simulink model "SPWM_tiaozhi"  (R2024b)
settings: Solver=VariableStepAuto  StartTime=1  StopTime=20  RelTol=1e-5  AbsTol=1e-5
libraries: fl_lib x9, nesl_utility x8, spsControlledVoltageSourceLib x3, ee_lib x3, spsPermanentMagnetSynchronousMachineLib x1, simulink x1, sps_lib x1
settings Model: SimulationMode=accelerator  Creator=刘炳宏  LastModifiedBy=刘炳宏
settings DataIOCC: ReturnWorkspaceOutputs=off

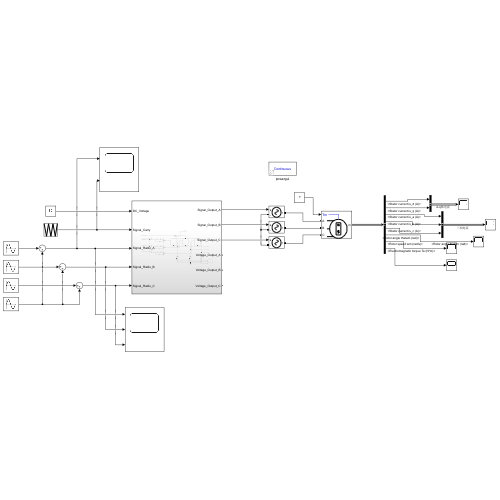
[thumbnail: Simulink's stored preview of the top-level diagram]
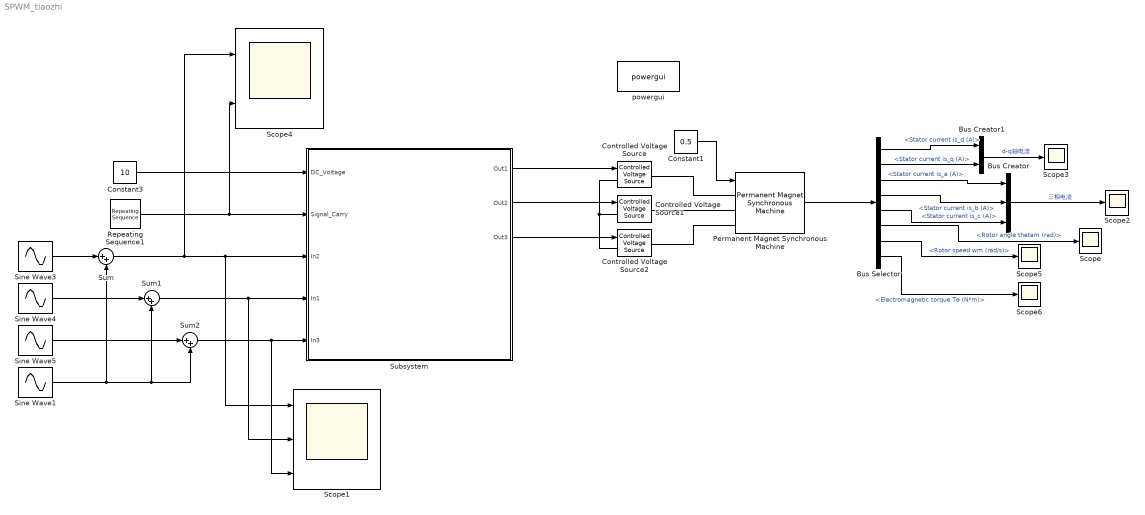
== system SPWM_tiaozhi ==
  Bus Creator : BusCreator  Inputs=3
  Bus Creator1 : BusCreator  Inputs=2
  Bus Selector : BusSelector  OutputSignals=Stator current is_d (A),Stator current is_q (A),Stator current is_a (A),Stator current is_b (A),Stator current is_c (A),Rotor angle thetam (rad),Rotor speed wm (rad/s),Electromagnetic torque Te (N*m)
  Constant1 : Constant  Value=0.5
  Constant3 : Constant  Value=10
  Controlled Voltage Source : spsControlledVoltageSourceLib/Controlled Voltage Source  Initialize=on  Source_Type=DC  Amplitude=0  Phase=0  Frequency=0  Measurements=None
  Controlled Voltage Source1 : spsControlledVoltageSourceLib/Controlled Voltage Source  Initialize=on  Source_Type=DC  Amplitude=0  Phase=0  Frequency=0  Measurements=None
  Controlled Voltage Source2 : spsControlledVoltageSourceLib/Controlled Voltage Source  Initialize=on  Source_Type=DC  Amplitude=0  Phase=0  Frequency=0  Measurements=None
  Permanent Magnet Synchronous Machine : spsPermanentMagnetSynchronousMachineLib/Permanent Magnet Synchronous Machine  NbPhases=3  FluxDistribution=Sinusoidal  RotorType=Round  MechanicalLoad=Torque Tm  PresetModel=No  ShowDetailedParameters=on  MeasurementBus=off  Resistance=0.18  Inductance=8.5e-3  dqInductances=[8.5e-3,8.5e-3]  La=8.5e-3  MachineConstant=Flux linkage established by magnets (V.s)  Flux=0.074147  VoltageCst=134.4878  TorqueCst=1.1122  Flat=120  Mechanical=[0.00062 0.0003505 10 0]  PolePairs=4  InitialConditions=[0,1, 0,0]  InitialConditions5ph=[0 0 0 0 0 0]  RefAngle=Aligned with phase A axis (original Park)  IterativeDiscreteModel=Trapezoidal non iterative  TsBlock=-1  TsPowergui=0
  Repeating Sequence1 : simulink/Sources/Repeating Sequence  rep_seq_t=[0,0.5/(5000),1/(5000)]  rep_seq_y=[1,-1,1]
  Scope{,2..3,5..6} (5 alike) : Scope
  Scope1 : Scope  NumInputPorts=3
  Scope4 : Scope  NumInputPorts=2
  Sine Wave1 : Sin  Amplitude=0.02*10  Frequency=6*3.14159*5*10  SampleTime=0
  Sine Wave3 : Sin  Amplitude=0.05*10  Frequency=2*3.14159*5*10  SampleTime=0
  Sine Wave4 : Sin  Amplitude=0.05*10  Frequency=2*3.14159*5*10  Phase=2*3.14159/3  SampleTime=0
  Sine Wave5 : Sin  Amplitude=0.05*10  Frequency=2*3.14159*5*10  Phase=-2*3.14159/3  SampleTime=0
  Subsystem : Subsystem
  Sum : Sum  Inputs=|++
  Sum1 : Sum  Inputs=|++
  Sum2 : Sum  Inputs=|++
  powergui : sps_lib/powergui  Priority=1  SimulationMode=Continuous  SampleTime=50e-6  frequency=60  Iterations=50  frequencyindice=0  Pbase=100e6  ErrMax=1e-4  UnitsV=kV  UnitsW=MW  buscounter=0  FunctionMessages=off  echomessages=off  EnableUseOfTLC=off  CurrentSourceSwitches=off  DisableSnubberDevices=off  DisableRonSwitches=off  DisableVfSwitches=off  DisplayEquations=off  AutomaticDiscreteSolvers=off  SolverType=Tustin/Backward Euler (TBE)  Interpol=off  ExternalGateDelay=off  methode=off  Ts=100  x0status=blocks  SPID=on  SwTol=0  HookPort=off  NonlinearTolerance=1e-4  nMaxIteration=100  ContinueOnMaxIteration=off  RestoreLinks=warning  ResistiveCurrentMeasurement=off  Frange=[0:2:500]  Ylog=off  Xlog=on  ShowGrid=off  save=off  variable=ZData  structure=0  ZoomFFT=off  StartTime=0.0  cycles=1  DisplayStyle=1  fundamental=60  FreqAxis=off  MaxFrequency=1000  frequencyindicesteady=1  RmsSteady=1  display=off
  wires:
  Repeating Sequence1/1 -> Scope4/2, Subsystem/2(Signal_Carry)
  Constant3/1 -> Subsystem/1(DC_Voltage)
  Sine Wave3/1 -> Sum/1
  Sum/1 -> Scope4/1, Scope1/1, Subsystem/3(In2)
  Sum1/1 -> Scope1/2, Subsystem/4(In1)
  Sine Wave4/1 -> Sum1/1
  Sine Wave1/1 -> Sum2/2, Sum1/2, Sum/2
  Sine Wave5/1 -> Sum2/1
  Sum2/1 -> Scope1/3, Subsystem/5(In3)
  Subsystem/1(Out1) -> Controlled Voltage Source/1
  Subsystem/3(Out3) -> Controlled Voltage Source2/1
  Subsystem/2(Out2) -> Controlled Voltage Source1/1
  Bus Selector/5 -> Bus Creator/3  "<Stator current is_c (A)>"
  Bus Selector/4 -> Bus Creator/2  "<Stator current is_b (A)>"
  Bus Selector/2 -> Bus Creator1/2  "<Stator current is_q (A)>"
  Bus Selector/1 -> Bus Creator1/1  "<Stator current is_d (A)>"
  Bus Creator1/1 -> Scope3/1  "d-q轴电流"
  Permanent Magnet Synchronous Machine/1 -> Bus Selector/1
  Bus Creator/1 -> Scope2/1  "三相电流"
  Bus Selector/3 -> Bus Creator/1  "<Stator current is_a (A)>"
  Bus Selector/6 -> Scope/1  "<Rotor angle thetam (rad)>"
  Bus Selector/7 -> Scope5/1  "<Rotor speed wm (rad/s)>"
  Bus Selector/8 -> Scope6/1  "<Electromagnetic torque Te (N*m)>"
  Constant1/1 -> Permanent Magnet Synchronous Machine/1
  connections:
  Controlled Voltage Source/LConn1 -- Controlled Voltage Source1/LConn1 -- Controlled Voltage Source2/LConn1
  Permanent Magnet Synchronous Machine/LConn2 -- Controlled Voltage Source1/RConn1
  Permanent Magnet Synchronous Machine/LConn1 -- Controlled Voltage Source/RConn1
  Permanent Magnet Synchronous Machine/LConn3 -- Controlled Voltage Source2/RConn1

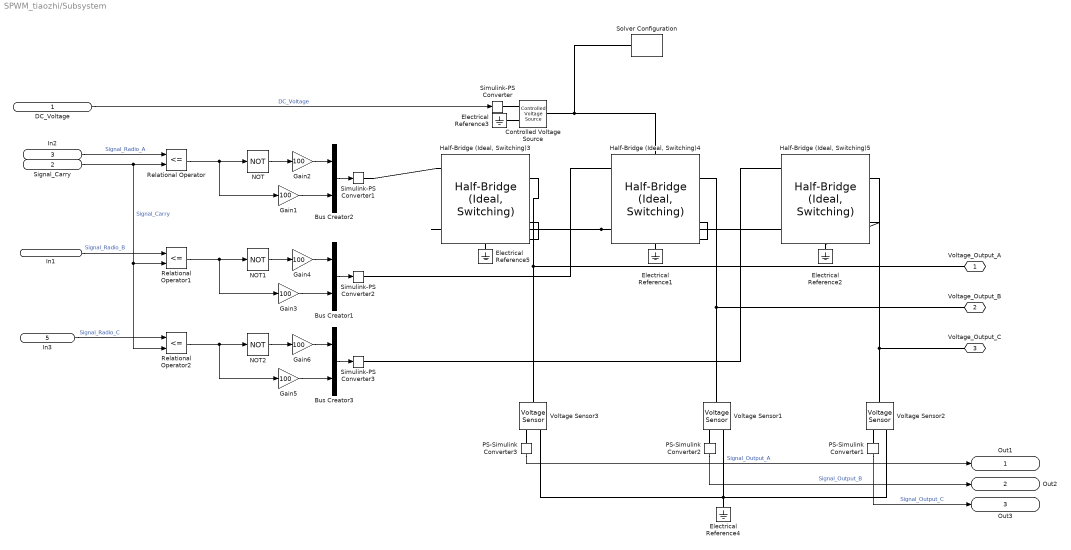
== system SPWM_tiaozhi/Subsystem ==
  DC_Voltage : Inport
  Signal_Carry : Inport  Port=2
  In2 : Inport  Port=3
  In1 : Inport  Port=4
  In3 : Inport  Port=5
  Bus Creator1 : BusCreator  Inputs=2
  Bus Creator2 : BusCreator  Inputs=2
  Bus Creator3 : BusCreator  Inputs=2
  Controlled Voltage Source : fl_lib/Electrical/Electrical Sources/Controlled Voltage Source
  Electrical Reference{1..5} (5 alike) : fl_lib/Electrical/Electrical Elements/Electrical Reference
  Gain{1..6} (6 alike) : Gain  Gain=100  OutDataTypeStr=double
  "Half-Bridge (Ideal, Switching)3" : ee_lib/Semiconductors & Converters/Half-Bridge (Ideal, Switching)  control_port=ee.enum.controlport.ps  device_type=ee.enum.converters.switches.mosfet  gto_Vgt=6 V  gto_Vgt_off=-1 V  gto_Ih=1 A  gto_thermal_loss_option=ee.enum.converters.thermalLossOption.constantvalues  gto_Vf=0.8 V  gto_Ron=0.001 Ohm  gto_Von_data=[0, .1, .6, .8, 1, 1.3, 1.6, 2, 2.4; 0, .1, .7, 1, 1.2, 1.5, 1.9, 2.4, 2.8] V  gto_Tj=[298.15, 398.15] K  gto_Iout_data=[0, .1, 1, 5, 10, 20, 40, 70, 100] A  igbt_Vth=6 V  igbt_thermal_loss_option=ee.enum.converters.thermalLossOption.constantvalues  igbt_Vf=0.8 V  igbt_Ron=0.001 Ohm  igbt_Von_data=[0, .1, .6, .8, 1, 1.3, 1.6, 2, 2.4; 0, .1, .7, 1, 1.2, 1.5, 1.9, 2.4, 2.8] V  igbt_Tj=[298.15, 398.15] K  igbt_Iout_data=[0, .1, 1, 5, 10, 20, 40, 70, 100] A  mosfet_Vth=2 V  mosfet_thermal_loss_option=ee.enum.converters.thermalLossOption.constantvalues  mosfet_Rds=0.01 Ohm  mosfet_Von_data=[0, 1.1, 1.3, 1.45, 1.75, 2.25, 2.7; 0, 1, 1.15, 1.35, 1.7, 2.35, 3] V  mosfet_Tj=[298.15, 398.15] K  mosfet_Iout_data=[0, 10, 50, 100, 200, 400, 600] A  Goff=1e-6 1/Ohm  gto_Eon_data=[0, .0024, .024, .12, .2, .48, 1.04, 2.16, 3.24; 0, .003, .03, .15, .25, .6, 1.3, 2.7, 4.05] * 1e-3 J  igbt_Eon_data=[0, .0024, .024, .12, .2, .48, 1.04, 2.16, 3.24; 0, .003, .03, .15, .25, .6, 1.3, 2.7, 4.05] * 1e-3 J  mosfet_Eon_data=[0, .29, 1.43, 2.86, 5.71, 13.14, 22.86; 0, .57, 2.63, 5.14, 10.29, 20.57, 30.29] * 1e-3 J  gto_Eoff_data=[0, .0007, .0066, .033, .066, .17, .33, .83, 1.5; 0, .001, .01, .05, .1, .25, .5, 1.2, 2.2] * 1e-3 J  igbt_Eoff_data=[0, .0007, .0066, .033, .066, .17, .33, .83, 1.5; 0, .001, .01, .05, .1, .25, .5, 1.2, 2.2] * 1e-3 J  mosfet_Eoff_data=[0, .21, 1.07, 2.14, 4.29, 9.86, 17.14; 0, .43, 1.97, 3.86, 7.71, 15.43, 22.71] * 1e-3 J  igbt_Eon_data_3D=[zeros(2, 9, 3)] J  mosfet_Eon_data_3D=[zeros(2, 7, 3)] J  igbt_Eoff_data_3D=[zeros(2, 9, 3)] J  mosfet_Eoff_data_3D=[zeros(2, 7, 3)] J  gto_Erec_data=[0, .0031, .021, .11, .21, .43, .99, 1.71, 3.078; 0, .0041, .043, .2, .39, .77, 1.54, 2.27, 4.08] * 1e-3 J  igbt_Erec_data=[0, .0031, .021, .11, .21, .43, .99, 1.71, 3.078; 0, .0041, .043, .2, .39, .77, 1.54, 2.27, 4.08] * 1e-3 J  mosfet_Erec_data=[0, .0031, .021, .11, .21, .43, .99; 0, .0041, .043, .2, .39, .77, 1.54] * 1e-3 J  gto_Tj_loss=[298.15, 398.15] K  igbt_Tj_loss=[298.15, 398.15] K  mosfet_Tj_loss=[298.15, 398.15] K  gto_Iout_data_loss=[0, .1, 1, 5, 10, 20, 40, 70, 100] A  igbt_Iout_data_loss=[0, .1, 1, 5, 10, 20, 40, 70, 100] A  mosfet_Iout_data_loss=[0, 10, 50, 100, 200, 400, 600] A  gto_Eon_scalar=22.86e-3 J  igbt_Eon_scalar=22.86e-3 J  mosfet_Eon_scalar=22.86e-3 J  gto_Eoff_scalar=17.14e-3 J  igbt_Eoff_scalar=17.14e-3 J  mosfet_Eoff_scalar=17.14e-3 J  gto_Erec_scalar=5.70e-3 J  igbt_Erec_scalar=5.70e-3 J  mosfet_Erec_scalar=5.70e-3 J  gto_Iout_scalar=600 A  igbt_Iout_scalar=600 A  mosfet_Iout_scalar=600 A  igbt_tabulateWithVce=false  mosfet_tabulateWithVds=false  igbt_Vce_loss=[0, 150, 300] V  mosfet_Vds_loss=[0, 150, 300] V  Voff=300 V  gto_Eoff_natural_commutation=10e-3 J  applySwLossToSupply=false  tauApplySwLoss=1e-3 s  diode_param=ee.enum.include.yes  diode_ModelType=ee.enum.converters.diodeModelType.pwl  diode_TableType=ee.enum.diode.tableType.IfMat  diode_ReverseIVType=ee.enum.diode.diodeReverseIV.constant  diode_IfMat=[.07, .12, .19, 1.75, 4.24, 7.32, 11.2; .16, .3, .72, 2.14, 4.02, 6.35, 9.12] A  diode_VfMat=[.9, 1.15, 1.25, 1.5, 1.75, 2.17, 2.6, 2.85; .58, .68, .75, 1.1, 1.38, 1.77, 2.27, 2.7] V  diode_TjVec=[25, 125] degC  diode_VfVec=[.5, .7, .9, 1.3, 1.7, 2.1, 2.5] V  diode_IfVec=[.1, .2, .5, 1, 2, 4, 7, 10] A  diode_IrMat=[1e-06, 2e-06, 5e-06, 1e-05, 2.5e-05, 5e-05, .0001; 2e-06, 5e-06, 1e-05, 4e-05, 8e-05, .0002, .0005] A  diode_VrMat=[10, 100, 200, 250, 300, 325, 350; 10, 70, 160, 220, 270, 300, 320] V  diode_VrVec=[10, 20, 40, 50, 70, 80, 100] V  diode_IrVec=[1e-06, 2e-06, 5e-06, 1e-05, 2e-05, 5e-05, .0001] A  diode_Vf=0.8 V  diode_Ron=0.001 Ohm  diode_Goff=1e-5 1/Ohm  separateThermalPort=false  separateThermalPortsForDiodes=false  thermal_network_parameterization=ee.enum.thermalNetworkTopology.external  thermal_mass_parameterization=ee.enum.thermalNetwork.timeconstant  Rth=[.03, .2] K/W  Rth_Cauer=[.03, .1, .2] K/W  Rth_Foster=[.08, .14, .22, .16] K/W  thermal_mass=[3, 25] J/K  thermal_mass_Cauer=[3, 10, 25] J/K  thermal_mass_Foster=[.001, .005, .05, .5] J/K  thermal_time_constant=[.1, 5] s  thermal_time_constant_Cauer=[.1, 1, 5] s  thermal_time_constant_Foster=[7e-05, .0007, .01, .08] s  thermal_mass_initial_temperatures=[25, 25] degC  thermal_mass_initial_temperatures_Cauer=[25, 25, 25] degC  junction_thermal_mass=0.1 J/K  Tvec_initial_Foster=[25, 25, 25, 25] degC  RthDiode=[.03, .2] K/W  RthCauerDiode=[.03, .1, .2] K/W  RthFosterDiode=[.08, .14, .22, .16] K/W  ThermalMassDiode=[3, 25] J/K  ThermalMassCauerDiode=[3, 10, 25] J/K  ThermalMassFosterDiode=[.001, .005, .05, .5] J/K  ThermalTauDiode=[.1, 5] s  ThermalTauCauerDiode=[.1, 1, 5] s  ThermalTauFosterDiode=[7e-05, .0007, .01, .08] s  ThermalMassInitTempDiode=[25, 25] degC  ThermalMassInitTempCauerDiode=[25, 25, 25] degC  JunctionThermalMassDiode=0.1 J/K  TVecInitialFosterDiode=[25, 25, 25, 25] degC  junction_temperature_specify=off  junction_temperature_priority=None  junction_temperature=25 degC  junction_temperature_nominal_specify=off  junction_temperature_nominal_value=1  junction_temperature_nominal_unit=degC  upperSwitchTemp_specify=off  upperSwitchTemp_priority=None  upperSwitchTemp=25 degC  upperSwitchTemp_nominal_specify=off  upperSwitchTemp_nominal_value=1  upperSwitchTemp_nominal_unit=degC  lowerSwitchTemp_specify=off  lowerSwitchTemp_priority=None  lowerSwitchTemp=25 degC  lowerSwitchTemp_nominal_specify=off  lowerSwitchTemp_nominal_value=1  lowerSwitchTemp_nominal_unit=degC  upperDiodeTemp_specify=off  upperDiodeTemp_priority=None  upperDiodeTemp=25 degC  upperDiodeTemp_nominal_specify=off  upperDiodeTemp_nominal_value=1  upperDiodeTemp_nominal_unit=degC  lowerDiodeTemp_specify=off  lowerDiodeTemp_priority=None  lowerDiodeTemp=25 degC  lowerDiodeTemp_nominal_specify=off  lowerDiodeTemp_nominal_value=1  lowerDiodeTemp_nominal_unit=degC
      settings: InternalSimscapePortConfiguration="{\"Bottom\":[{\"id\":\"n\",\"label\":\"-\",\"type\":\"foundation.electrical.electrical\"}],\"Left\":[{\"id\":\"G\",\"label\":\"G\",\"type\":\"input\"},{\"id\":\"H\",\"label\":\"H\",\"type\":\"foundation.thermal.thermal\"}],\"Right\":[{\"id\":\"o\",\"label\":\"o\",\"type\":\"foundation.electrical.electrical\"}],\"Top\":[{\"id\":\"p\",\"label\":\"+\",\"type\":\"foundation.electrical.electrical\"}]}"
  "Half-Bridge (Ideal, Switching)4" : ee_lib/Semiconductors & Converters/Half-Bridge (Ideal, Switching)  control_port=ee.enum.controlport.ps  device_type=ee.enum.converters.switches.mosfet  gto_Vgt=6 V  gto_Vgt_off=-1 V  gto_Ih=1 A  gto_thermal_loss_option=ee.enum.converters.thermalLossOption.constantvalues  gto_Vf=0.8 V  gto_Ron=0.001 Ohm  gto_Von_data=[0, .1, .6, .8, 1, 1.3, 1.6, 2, 2.4; 0, .1, .7, 1, 1.2, 1.5, 1.9, 2.4, 2.8] V  gto_Tj=[298.15, 398.15] K  gto_Iout_data=[0, .1, 1, 5, 10, 20, 40, 70, 100] A  igbt_Vth=6 V  igbt_thermal_loss_option=ee.enum.converters.thermalLossOption.constantvalues  igbt_Vf=0.8 V  igbt_Ron=0.001 Ohm  igbt_Von_data=[0, .1, .6, .8, 1, 1.3, 1.6, 2, 2.4; 0, .1, .7, 1, 1.2, 1.5, 1.9, 2.4, 2.8] V  igbt_Tj=[298.15, 398.15] K  igbt_Iout_data=[0, .1, 1, 5, 10, 20, 40, 70, 100] A  mosfet_Vth=2 V  mosfet_thermal_loss_option=ee.enum.converters.thermalLossOption.constantvalues  mosfet_Rds=0.01 Ohm  mosfet_Von_data=[0, 1.1, 1.3, 1.45, 1.75, 2.25, 2.7; 0, 1, 1.15, 1.35, 1.7, 2.35, 3] V  mosfet_Tj=[298.15, 398.15] K  mosfet_Iout_data=[0, 10, 50, 100, 200, 400, 600] A  Goff=1e-6 1/Ohm  gto_Eon_data=[0, .0024, .024, .12, .2, .48, 1.04, 2.16, 3.24; 0, .003, .03, .15, .25, .6, 1.3, 2.7, 4.05] * 1e-3 J  igbt_Eon_data=[0, .0024, .024, .12, .2, .48, 1.04, 2.16, 3.24; 0, .003, .03, .15, .25, .6, 1.3, 2.7, 4.05] * 1e-3 J  mosfet_Eon_data=[0, .29, 1.43, 2.86, 5.71, 13.14, 22.86; 0, .57, 2.63, 5.14, 10.29, 20.57, 30.29] * 1e-3 J  gto_Eoff_data=[0, .0007, .0066, .033, .066, .17, .33, .83, 1.5; 0, .001, .01, .05, .1, .25, .5, 1.2, 2.2] * 1e-3 J  igbt_Eoff_data=[0, .0007, .0066, .033, .066, .17, .33, .83, 1.5; 0, .001, .01, .05, .1, .25, .5, 1.2, 2.2] * 1e-3 J  mosfet_Eoff_data=[0, .21, 1.07, 2.14, 4.29, 9.86, 17.14; 0, .43, 1.97, 3.86, 7.71, 15.43, 22.71] * 1e-3 J  igbt_Eon_data_3D=[zeros(2, 9, 3)] J  mosfet_Eon_data_3D=[zeros(2, 7, 3)] J  igbt_Eoff_data_3D=[zeros(2, 9, 3)] J  mosfet_Eoff_data_3D=[zeros(2, 7, 3)] J  gto_Erec_data=[0, .0031, .021, .11, .21, .43, .99, 1.71, 3.078; 0, .0041, .043, .2, .39, .77, 1.54, 2.27, 4.08] * 1e-3 J  igbt_Erec_data=[0, .0031, .021, .11, .21, .43, .99, 1.71, 3.078; 0, .0041, .043, .2, .39, .77, 1.54, 2.27, 4.08] * 1e-3 J  mosfet_Erec_data=[0, .0031, .021, .11, .21, .43, .99; 0, .0041, .043, .2, .39, .77, 1.54] * 1e-3 J  gto_Tj_loss=[298.15, 398.15] K  igbt_Tj_loss=[298.15, 398.15] K  mosfet_Tj_loss=[298.15, 398.15] K  gto_Iout_data_loss=[0, .1, 1, 5, 10, 20, 40, 70, 100] A  igbt_Iout_data_loss=[0, .1, 1, 5, 10, 20, 40, 70, 100] A  mosfet_Iout_data_loss=[0, 10, 50, 100, 200, 400, 600] A  gto_Eon_scalar=22.86e-3 J  igbt_Eon_scalar=22.86e-3 J  mosfet_Eon_scalar=22.86e-3 J  gto_Eoff_scalar=17.14e-3 J  igbt_Eoff_scalar=17.14e-3 J  mosfet_Eoff_scalar=17.14e-3 J  gto_Erec_scalar=5.70e-3 J  igbt_Erec_scalar=5.70e-3 J  mosfet_Erec_scalar=5.70e-3 J  gto_Iout_scalar=600 A  igbt_Iout_scalar=600 A  mosfet_Iout_scalar=600 A  igbt_tabulateWithVce=false  mosfet_tabulateWithVds=false  igbt_Vce_loss=[0, 150, 300] V  mosfet_Vds_loss=[0, 150, 300] V  Voff=300 V  gto_Eoff_natural_commutation=10e-3 J  applySwLossToSupply=false  tauApplySwLoss=1e-3 s  diode_param=ee.enum.include.yes  diode_ModelType=ee.enum.converters.diodeModelType.pwl  diode_TableType=ee.enum.diode.tableType.IfMat  diode_ReverseIVType=ee.enum.diode.diodeReverseIV.constant  diode_IfMat=[.07, .12, .19, 1.75, 4.24, 7.32, 11.2; .16, .3, .72, 2.14, 4.02, 6.35, 9.12] A  diode_VfMat=[.9, 1.15, 1.25, 1.5, 1.75, 2.17, 2.6, 2.85; .58, .68, .75, 1.1, 1.38, 1.77, 2.27, 2.7] V  diode_TjVec=[25, 125] degC  diode_VfVec=[.5, .7, .9, 1.3, 1.7, 2.1, 2.5] V  diode_IfVec=[.1, .2, .5, 1, 2, 4, 7, 10] A  diode_IrMat=[1e-06, 2e-06, 5e-06, 1e-05, 2.5e-05, 5e-05, .0001; 2e-06, 5e-06, 1e-05, 4e-05, 8e-05, .0002, .0005] A  diode_VrMat=[10, 100, 200, 250, 300, 325, 350; 10, 70, 160, 220, 270, 300, 320] V  diode_VrVec=[10, 20, 40, 50, 70, 80, 100] V  diode_IrVec=[1e-06, 2e-06, 5e-06, 1e-05, 2e-05, 5e-05, .0001] A  diode_Vf=0.8 V  diode_Ron=0.001 Ohm  diode_Goff=1e-5 1/Ohm  separateThermalPort=false  separateThermalPortsForDiodes=false  thermal_network_parameterization=ee.enum.thermalNetworkTopology.external  thermal_mass_parameterization=ee.enum.thermalNetwork.timeconstant  Rth=[.03, .2] K/W  Rth_Cauer=[.03, .1, .2] K/W  Rth_Foster=[.08, .14, .22, .16] K/W  thermal_mass=[3, 25] J/K  thermal_mass_Cauer=[3, 10, 25] J/K  thermal_mass_Foster=[.001, .005, .05, .5] J/K  thermal_time_constant=[.1, 5] s  thermal_time_constant_Cauer=[.1, 1, 5] s  thermal_time_constant_Foster=[7e-05, .0007, .01, .08] s  thermal_mass_initial_temperatures=[25, 25] degC  thermal_mass_initial_temperatures_Cauer=[25, 25, 25] degC  junction_thermal_mass=0.1 J/K  Tvec_initial_Foster=[25, 25, 25, 25] degC  RthDiode=[.03, .2] K/W  RthCauerDiode=[.03, .1, .2] K/W  RthFosterDiode=[.08, .14, .22, .16] K/W  ThermalMassDiode=[3, 25] J/K  ThermalMassCauerDiode=[3, 10, 25] J/K  ThermalMassFosterDiode=[.001, .005, .05, .5] J/K  ThermalTauDiode=[.1, 5] s  ThermalTauCauerDiode=[.1, 1, 5] s  ThermalTauFosterDiode=[7e-05, .0007, .01, .08] s  ThermalMassInitTempDiode=[25, 25] degC  ThermalMassInitTempCauerDiode=[25, 25, 25] degC  JunctionThermalMassDiode=0.1 J/K  TVecInitialFosterDiode=[25, 25, 25, 25] degC  junction_temperature_specify=off  junction_temperature_priority=None  junction_temperature=25 degC  junction_temperature_nominal_specify=off  junction_temperature_nominal_value=1  junction_temperature_nominal_unit=degC  upperSwitchTemp_specify=off  upperSwitchTemp_priority=None  upperSwitchTemp=25 degC  upperSwitchTemp_nominal_specify=off  upperSwitchTemp_nominal_value=1  upperSwitchTemp_nominal_unit=degC  lowerSwitchTemp_specify=off  lowerSwitchTemp_priority=None  lowerSwitchTemp=25 degC  lowerSwitchTemp_nominal_specify=off  lowerSwitchTemp_nominal_value=1  lowerSwitchTemp_nominal_unit=degC  upperDiodeTemp_specify=off  upperDiodeTemp_priority=None  upperDiodeTemp=25 degC  upperDiodeTemp_nominal_specify=off  upperDiodeTemp_nominal_value=1  upperDiodeTemp_nominal_unit=degC  lowerDiodeTemp_specify=off  lowerDiodeTemp_priority=None  lowerDiodeTemp=25 degC  lowerDiodeTemp_nominal_specify=off  lowerDiodeTemp_nominal_value=1  lowerDiodeTemp_nominal_unit=degC
      settings: InternalSimscapePortConfiguration="{\"Bottom\":[{\"id\":\"n\",\"label\":\"-\",\"type\":\"foundation.electrical.electrical\"}],\"Left\":[{\"id\":\"G\",\"label\":\"G\",\"type\":\"input\"},{\"id\":\"H\",\"label\":\"H\",\"type\":\"foundation.thermal.thermal\"}],\"Right\":[{\"id\":\"o\",\"label\":\"o\",\"type\":\"foundation.electrical.electrical\"}],\"Top\":[{\"id\":\"p\",\"label\":\"+\",\"type\":\"foundation.electrical.electrical\"}]}"
  "Half-Bridge (Ideal, Switching)5" : ee_lib/Semiconductors & Converters/Half-Bridge (Ideal, Switching)  control_port=ee.enum.controlport.ps  device_type=ee.enum.converters.switches.mosfet  gto_Vgt=6 V  gto_Vgt_off=-1 V  gto_Ih=1 A  gto_thermal_loss_option=ee.enum.converters.thermalLossOption.constantvalues  gto_Vf=0.8 V  gto_Ron=0.001 Ohm  gto_Von_data=[0, .1, .6, .8, 1, 1.3, 1.6, 2, 2.4; 0, .1, .7, 1, 1.2, 1.5, 1.9, 2.4, 2.8] V  gto_Tj=[298.15, 398.15] K  gto_Iout_data=[0, .1, 1, 5, 10, 20, 40, 70, 100] A  igbt_Vth=6 V  igbt_thermal_loss_option=ee.enum.converters.thermalLossOption.constantvalues  igbt_Vf=0.8 V  igbt_Ron=0.001 Ohm  igbt_Von_data=[0, .1, .6, .8, 1, 1.3, 1.6, 2, 2.4; 0, .1, .7, 1, 1.2, 1.5, 1.9, 2.4, 2.8] V  igbt_Tj=[298.15, 398.15] K  igbt_Iout_data=[0, .1, 1, 5, 10, 20, 40, 70, 100] A  mosfet_Vth=2 V  mosfet_thermal_loss_option=ee.enum.converters.thermalLossOption.constantvalues  mosfet_Rds=0.01 Ohm  mosfet_Von_data=[0, 1.1, 1.3, 1.45, 1.75, 2.25, 2.7; 0, 1, 1.15, 1.35, 1.7, 2.35, 3] V  mosfet_Tj=[298.15, 398.15] K  mosfet_Iout_data=[0, 10, 50, 100, 200, 400, 600] A  Goff=1e-6 1/Ohm  gto_Eon_data=[0, .0024, .024, .12, .2, .48, 1.04, 2.16, 3.24; 0, .003, .03, .15, .25, .6, 1.3, 2.7, 4.05] * 1e-3 J  igbt_Eon_data=[0, .0024, .024, .12, .2, .48, 1.04, 2.16, 3.24; 0, .003, .03, .15, .25, .6, 1.3, 2.7, 4.05] * 1e-3 J  mosfet_Eon_data=[0, .29, 1.43, 2.86, 5.71, 13.14, 22.86; 0, .57, 2.63, 5.14, 10.29, 20.57, 30.29] * 1e-3 J  gto_Eoff_data=[0, .0007, .0066, .033, .066, .17, .33, .83, 1.5; 0, .001, .01, .05, .1, .25, .5, 1.2, 2.2] * 1e-3 J  igbt_Eoff_data=[0, .0007, .0066, .033, .066, .17, .33, .83, 1.5; 0, .001, .01, .05, .1, .25, .5, 1.2, 2.2] * 1e-3 J  mosfet_Eoff_data=[0, .21, 1.07, 2.14, 4.29, 9.86, 17.14; 0, .43, 1.97, 3.86, 7.71, 15.43, 22.71] * 1e-3 J  igbt_Eon_data_3D=[zeros(2, 9, 3)] J  mosfet_Eon_data_3D=[zeros(2, 7, 3)] J  igbt_Eoff_data_3D=[zeros(2, 9, 3)] J  mosfet_Eoff_data_3D=[zeros(2, 7, 3)] J  gto_Erec_data=[0, .0031, .021, .11, .21, .43, .99, 1.71, 3.078; 0, .0041, .043, .2, .39, .77, 1.54, 2.27, 4.08] * 1e-3 J  igbt_Erec_data=[0, .0031, .021, .11, .21, .43, .99, 1.71, 3.078; 0, .0041, .043, .2, .39, .77, 1.54, 2.27, 4.08] * 1e-3 J  mosfet_Erec_data=[0, .0031, .021, .11, .21, .43, .99; 0, .0041, .043, .2, .39, .77, 1.54] * 1e-3 J  gto_Tj_loss=[298.15, 398.15] K  igbt_Tj_loss=[298.15, 398.15] K  mosfet_Tj_loss=[298.15, 398.15] K  gto_Iout_data_loss=[0, .1, 1, 5, 10, 20, 40, 70, 100] A  igbt_Iout_data_loss=[0, .1, 1, 5, 10, 20, 40, 70, 100] A  mosfet_Iout_data_loss=[0, 10, 50, 100, 200, 400, 600] A  gto_Eon_scalar=22.86e-3 J  igbt_Eon_scalar=22.86e-3 J  mosfet_Eon_scalar=22.86e-3 J  gto_Eoff_scalar=17.14e-3 J  igbt_Eoff_scalar=17.14e-3 J  mosfet_Eoff_scalar=17.14e-3 J  gto_Erec_scalar=5.70e-3 J  igbt_Erec_scalar=5.70e-3 J  mosfet_Erec_scalar=5.70e-3 J  gto_Iout_scalar=600 A  igbt_Iout_scalar=600 A  mosfet_Iout_scalar=600 A  igbt_tabulateWithVce=false  mosfet_tabulateWithVds=false  igbt_Vce_loss=[0, 150, 300] V  mosfet_Vds_loss=[0, 150, 300] V  Voff=300 V  gto_Eoff_natural_commutation=10e-3 J  applySwLossToSupply=false  tauApplySwLoss=1e-3 s  diode_param=ee.enum.include.yes  diode_ModelType=ee.enum.converters.diodeModelType.pwl  diode_TableType=ee.enum.diode.tableType.IfMat  diode_ReverseIVType=ee.enum.diode.diodeReverseIV.constant  diode_IfMat=[.07, .12, .19, 1.75, 4.24, 7.32, 11.2; .16, .3, .72, 2.14, 4.02, 6.35, 9.12] A  diode_VfMat=[.9, 1.15, 1.25, 1.5, 1.75, 2.17, 2.6, 2.85; .58, .68, .75, 1.1, 1.38, 1.77, 2.27, 2.7] V  diode_TjVec=[25, 125] degC  diode_VfVec=[.5, .7, .9, 1.3, 1.7, 2.1, 2.5] V  diode_IfVec=[.1, .2, .5, 1, 2, 4, 7, 10] A  diode_IrMat=[1e-06, 2e-06, 5e-06, 1e-05, 2.5e-05, 5e-05, .0001; 2e-06, 5e-06, 1e-05, 4e-05, 8e-05, .0002, .0005] A  diode_VrMat=[10, 100, 200, 250, 300, 325, 350; 10, 70, 160, 220, 270, 300, 320] V  diode_VrVec=[10, 20, 40, 50, 70, 80, 100] V  diode_IrVec=[1e-06, 2e-06, 5e-06, 1e-05, 2e-05, 5e-05, .0001] A  diode_Vf=0.8 V  diode_Ron=0.001 Ohm  diode_Goff=1e-5 1/Ohm  separateThermalPort=false  separateThermalPortsForDiodes=false  thermal_network_parameterization=ee.enum.thermalNetworkTopology.external  thermal_mass_parameterization=ee.enum.thermalNetwork.timeconstant  Rth=[.03, .2] K/W  Rth_Cauer=[.03, .1, .2] K/W  Rth_Foster=[.08, .14, .22, .16] K/W  thermal_mass=[3, 25] J/K  thermal_mass_Cauer=[3, 10, 25] J/K  thermal_mass_Foster=[.001, .005, .05, .5] J/K  thermal_time_constant=[.1, 5] s  thermal_time_constant_Cauer=[.1, 1, 5] s  thermal_time_constant_Foster=[7e-05, .0007, .01, .08] s  thermal_mass_initial_temperatures=[25, 25] degC  thermal_mass_initial_temperatures_Cauer=[25, 25, 25] degC  junction_thermal_mass=0.1 J/K  Tvec_initial_Foster=[25, 25, 25, 25] degC  RthDiode=[.03, .2] K/W  RthCauerDiode=[.03, .1, .2] K/W  RthFosterDiode=[.08, .14, .22, .16] K/W  ThermalMassDiode=[3, 25] J/K  ThermalMassCauerDiode=[3, 10, 25] J/K  ThermalMassFosterDiode=[.001, .005, .05, .5] J/K  ThermalTauDiode=[.1, 5] s  ThermalTauCauerDiode=[.1, 1, 5] s  ThermalTauFosterDiode=[7e-05, .0007, .01, .08] s  ThermalMassInitTempDiode=[25, 25] degC  ThermalMassInitTempCauerDiode=[25, 25, 25] degC  JunctionThermalMassDiode=0.1 J/K  TVecInitialFosterDiode=[25, 25, 25, 25] degC  junction_temperature_specify=off  junction_temperature_priority=None  junction_temperature=25 degC  junction_temperature_nominal_specify=off  junction_temperature_nominal_value=1  junction_temperature_nominal_unit=degC  upperSwitchTemp_specify=off  upperSwitchTemp_priority=None  upperSwitchTemp=25 degC  upperSwitchTemp_nominal_specify=off  upperSwitchTemp_nominal_value=1  upperSwitchTemp_nominal_unit=degC  lowerSwitchTemp_specify=off  lowerSwitchTemp_priority=None  lowerSwitchTemp=25 degC  lowerSwitchTemp_nominal_specify=off  lowerSwitchTemp_nominal_value=1  lowerSwitchTemp_nominal_unit=degC  upperDiodeTemp_specify=off  upperDiodeTemp_priority=None  upperDiodeTemp=25 degC  upperDiodeTemp_nominal_specify=off  upperDiodeTemp_nominal_value=1  upperDiodeTemp_nominal_unit=degC  lowerDiodeTemp_specify=off  lowerDiodeTemp_priority=None  lowerDiodeTemp=25 degC  lowerDiodeTemp_nominal_specify=off  lowerDiodeTemp_nominal_value=1  lowerDiodeTemp_nominal_unit=degC
      settings: InternalSimscapePortConfiguration="{\"Bottom\":[{\"id\":\"n\",\"label\":\"-\",\"type\":\"foundation.electrical.electrical\"}],\"Left\":[{\"id\":\"G\",\"label\":\"G\",\"type\":\"input\"},{\"id\":\"H\",\"label\":\"H\",\"type\":\"foundation.thermal.thermal\"}],\"Right\":[{\"id\":\"o\",\"label\":\"o\",\"type\":\"foundation.electrical.electrical\"}],\"Top\":[{\"id\":\"p\",\"label\":\"+\",\"type\":\"foundation.electrical.electrical\"}]}"
  NOT : Logic  Operator=NOT  IconShape=distinctive  AllPortsSameDT=off  OutDataTypeStr=boolean
  NOT1 : Logic  Operator=NOT  IconShape=distinctive  AllPortsSameDT=off  OutDataTypeStr=boolean
  NOT2 : Logic  Operator=NOT  IconShape=distinctive  AllPortsSameDT=off  OutDataTypeStr=boolean
  PS-Simulink Converter1 : nesl_utility/PS-Simulink Converter  PhysicalDomain=network_engine_domain  SubClassName=ps_output  LeftPortType=input  RightPortType=output  PseudoPeriodic=off  Frequencies=[]  VectorFormat=inherit  Unit=inherit  AffineConversion=off
  PS-Simulink Converter2 : nesl_utility/PS-Simulink Converter  PhysicalDomain=network_engine_domain  SubClassName=ps_output  LeftPortType=input  RightPortType=output  PseudoPeriodic=off  Frequencies=[]  VectorFormat=inherit  Unit=inherit  AffineConversion=off
  PS-Simulink Converter3 : nesl_utility/PS-Simulink Converter  PhysicalDomain=network_engine_domain  SubClassName=ps_output  LeftPortType=input  RightPortType=output  PseudoPeriodic=off  Frequencies=[]  VectorFormat=inherit  Unit=inherit  AffineConversion=off
  Relational Operator : RelationalOperator  Operator=<=  OutDataTypeStr=boolean  RndMeth=Simplest  InputSameDT=off
  Relational Operator1 : RelationalOperator  Operator=<=  OutDataTypeStr=boolean  RndMeth=Simplest  InputSameDT=off
  Relational Operator2 : RelationalOperator  Operator=<=  OutDataTypeStr=boolean  RndMeth=Simplest  InputSameDT=off
  Simulink-PS Converter{,1..3} (4 alike) : nesl_utility/Simulink-PS Converter  PhysicalDomain=network_engine_domain  SubClassName=ps_input  LeftPortType=input  RightPortType=output  PseudoPeriodic=off  Frequencies=[]  NoiseDistribution=none  NoiseParameters=[]  Unit=1  AffineConversion=off  FilteringAndDerivatives=provide  SimscapeFilterOrder=1  InputFilterTimeConstant=0.001  UdotUserProvided=0
  Solver Configuration : nesl_utility/Solver Configuration  PhysicalDomain=network_engine_domain  SubClassName=solver  LeftPortType=input  RightPortType=generic  Tones=[]  Harmonics=[]  SimulateNoise=off  Profile=off  UseLocalSampling=off  EnableSwitchedLinearOptims=on  FrequencyDomain=off  UseCCode=off  RelTol=0.001  AbsTol=0.001  MinStep=1e-09  ToWorkspace=off  RevertToSquareIcSolve=off  NumHomotopyIterations=100  PhasorMode=off  PhasorModeNumHarmonics=1  ConsistencySolver=NEWTON_XTOL_AFTER_FTOL  IndexReductionMethod=DerivativeReplacement  DoDC=off  ResidualTolerance=1e-09  ConsistencyTolSource=GLOBAL  ConsistencyAbsTol=0.001  ConsistencyRelTol=0.001  ConsistencyTolFactor=0.001  UseLocalSolver=off  LocalSolverChoice=NE_BACKWARD_EULER_ADVANCER  ResolveIndetEquations=on  FunctionEvalNumThread=1  LocalSolverSampleTime=0.001  DoFixedCost=off  MaxNonlinIter=3  MaxModeIter=2  ComputeImpulses=off  ImpulseIterations=2  LinearAlgebra=auto  LinearAlgebraNumThread=0  EquationFormulation=NE_TIME_EF  DelaysMemoryBudget=1024  AutomaticFiltering=on  FilteringTimeConstant=0.001  PartitionStorageMethod=AS_NEEDED  PartitionMemoryBudget=1024  PartitionMethod=ROBUST  MultibodyUseLocalSolver=off  MultibodyLocalSolverChoice=ODE1  MultibodyLocalSolverSampleTime=0.001
  Voltage Sensor1 : fl_lib/Electrical/Electrical Sensors/Voltage Sensor
  Voltage Sensor2 : fl_lib/Electrical/Electrical Sensors/Voltage Sensor
  Voltage Sensor3 : fl_lib/Electrical/Electrical Sensors/Voltage Sensor
  Voltage_Output_A : PMIOPort  Side=Right
  Voltage_Output_B : PMIOPort  Port=2  Side=Right
  Voltage_Output_C : PMIOPort  Port=3  Side=Right
  Out1 : Outport
  Out2 : Outport  Port=2
  Out3 : Outport  Port=3
  wires:
  DC_Voltage/1 -> Simulink-PS Converter/1  "DC_Voltage"
  NOT/1 -> Gain2/1
  Relational Operator/1 -> Gain1/1, NOT/1
  Gain2/1 -> Bus Creator2/1
  Gain1/1 -> Bus Creator2/2
  Bus Creator2/1 -> Simulink-PS Converter1/1
  Signal_Carry/1 -> Relational Operator1/2, Relational Operator2/2, Relational Operator/2  "Signal_Carry"
  In2/1 -> Relational Operator/1  "Signal_Radio_A"
  Relational Operator1/1 -> Gain3/1, NOT1/1
  NOT1/1 -> Gain4/1
  Gain4/1 -> Bus Creator1/1
  Bus Creator1/1 -> Simulink-PS Converter2/1
  Gain3/1 -> Bus Creator1/2
  Relational Operator2/1 -> Gain5/1, NOT2/1
  NOT2/1 -> Gain6/1
  Gain6/1 -> Bus Creator3/1
  Bus Creator3/1 -> Simulink-PS Converter3/1
  Gain5/1 -> Bus Creator3/2
  In1/1 -> Relational Operator1/1  "Signal_Radio_B"
  In3/1 -> Relational Operator2/1  "Signal_Radio_C"
  PS-Simulink Converter3/1 -> Out1/1  "Signal_Output_A"
  PS-Simulink Converter2/1 -> Out2/1  "Signal_Output_B"
  PS-Simulink Converter1/1 -> Out3/1  "Signal_Output_C"
  connections:
  Electrical Reference5/LConn1 -- "Half-Bridge (Ideal, Switching)3"/RConn2
  Electrical Reference1/LConn1 -- "Half-Bridge (Ideal, Switching)4"/RConn2
  "Half-Bridge (Ideal, Switching)5"/RConn2 -- Electrical Reference2/LConn1
  "Half-Bridge (Ideal, Switching)3"/LConn3 -- Solver Configuration/RConn1 -- Controlled Voltage Source/LConn1 -- "Half-Bridge (Ideal, Switching)5"/LConn3 -- "Half-Bridge (Ideal, Switching)4"/LConn3
  Electrical Reference3/LConn1 -- Controlled Voltage Source/RConn2
  Simulink-PS Converter/RConn1 -- Controlled Voltage Source/RConn1
  Simulink-PS Converter1/RConn1 -- "Half-Bridge (Ideal, Switching)3"/LConn1
  Simulink-PS Converter2/RConn1 -- "Half-Bridge (Ideal, Switching)4"/LConn1
  Simulink-PS Converter3/RConn1 -- "Half-Bridge (Ideal, Switching)5"/LConn1
  Voltage Sensor3/LConn1 -- Voltage_Output_A/RConn1 -- "Half-Bridge (Ideal, Switching)3"/RConn1
  Voltage Sensor1/LConn1 -- Voltage_Output_B/RConn1 -- "Half-Bridge (Ideal, Switching)4"/RConn1
  Voltage Sensor2/LConn1 -- Voltage_Output_C/RConn1 -- "Half-Bridge (Ideal, Switching)5"/RConn1
  Electrical Reference4/LConn1 -- Voltage Sensor3/RConn2 -- Voltage Sensor1/RConn2 -- Voltage Sensor2/RConn2
  PS-Simulink Converter1/LConn1 -- Voltage Sensor2/RConn1
  PS-Simulink Converter2/LConn1 -- Voltage Sensor1/RConn1
  PS-Simulink Converter3/LConn1 -- Voltage Sensor3/RConn1
